simulink model "twolinkDynamics"  (R2017b)
settings: Solver=VariableStepAuto  StartTime=0.0  StopTime=360  RelTol=1e-3
libraries: simulink x1
settings Model: SimulationMode=accelerator  Creator=ArsalanBangash  LastModifiedBy=ArsalanBangash

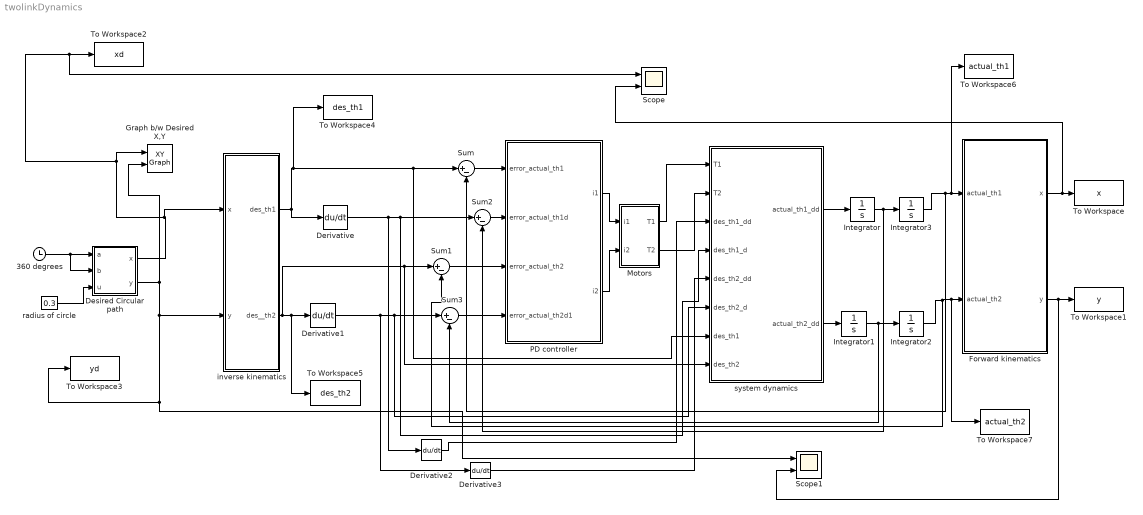
== system twolinkDynamics ==
  360 degrees : Clock
      settings: Decimation=360
  Derivative{,1..3} (4 alike) : Derivative
  Desired Circular path : MATLAB Function  TreatAsAtomicUnit=on
  "Forward kinematics " : MATLAB Function  TreatAsAtomicUnit=on
  Graph b/w Desired X,Y : simulink/Sinks/XY Graph  xmin=0  xmax=2  ymin=0  ymax=2  st=1
  Integrator{,1..3} (4 alike) : Integrator
  "Motors " : MATLAB Function  TreatAsAtomicUnit=on
  PD controller : Subsystem
  Scope : Scope  NumInputPorts=2
  Scope1 : Scope  NumInputPorts=2
  Sum{,1..3} (4 alike) : Sum  Inputs=|+-
  To Workspace : ToWorkspace  VariableName=x  SampleTime=1
  To Workspace1 : ToWorkspace  VariableName=y  SampleTime=1
  To Workspace2 : ToWorkspace  VariableName=xd  SampleTime=-1
  To Workspace3 : ToWorkspace  VariableName=yd  SampleTime=-1
  To Workspace4 : ToWorkspace  VariableName=des_th1  SampleTime=-1
  To Workspace5 : ToWorkspace  VariableName=des_th2  SampleTime=-1
  To Workspace6 : ToWorkspace  VariableName=actual_th1  SampleTime=-1
  To Workspace7 : ToWorkspace  VariableName=actual_th2  SampleTime=-1
  inverse kinematics : MATLAB Function  TreatAsAtomicUnit=on
  radius of circle : Constant  Value=0.3
  system dynamics : MATLAB Function  TreatAsAtomicUnit=on
  wires:
  360 degrees/1 -> Desired Circular path/2(b), Desired Circular path/1(a)
  radius of circle/1 -> Desired Circular path/3(u)
  Desired Circular path/1(x) -> Scope/1, To Workspace2/1, Graph b/w Desired X,Y/1, inverse kinematics/1(x)
  inverse kinematics/1(des_th1) -> To Workspace4/1, system dynamics/7(des_th1), Sum/1, Derivative/1
  "Motors "/1(T1) -> system dynamics/1(T1)
  "Forward kinematics "/1(x) -> Scope/2, To Workspace/1
  "Forward kinematics "/2(y) -> Scope1/2, To Workspace1/1
  Sum/1 -> PD controller/1(error_actual_th1)
  Sum2/1 -> PD controller/2(error_actual_th1d)
  PD controller/1(i1) -> "Motors "/1(i1)
  PD controller/2(i2) -> "Motors "/2(i2)
  "Motors "/2(T2) -> system dynamics/2(T2)
  Sum1/1 -> PD controller/3(error_actual_th2)
  Sum3/1 -> PD controller/4(error_actual_th2d1)
  system dynamics/1(actual_th1_dd) -> Integrator/1
  Integrator/1 -> Sum2/2, Integrator3/1
  Integrator3/1 -> Sum/2, To Workspace6/1, "Forward kinematics "/1(actual_th1)
  system dynamics/2(actual_th2_dd) -> Integrator1/1
  Integrator1/1 -> Integrator2/1, Sum3/2
  Integrator2/1 -> To Workspace7/1, "Forward kinematics "/2(actual_th2), Sum1/2
  inverse kinematics/2(des__th2) -> To Workspace5/1, Derivative1/1, system dynamics/8(des_th2), Sum1/1
  Derivative/1 -> system dynamics/4(des_th1_d), Sum2/1, Derivative2/1
  Derivative3/1 -> system dynamics/5(des_th2_dd)
  Derivative2/1 -> system dynamics/3(des_th1_dd)
  Derivative1/1 -> Derivative3/1, system dynamics/6(des_th2_d), Sum3/1
  Desired Circular path/2(y) -> Scope1/1, To Workspace3/1, inverse kinematics/2(y), Graph b/w Desired X,Y/2

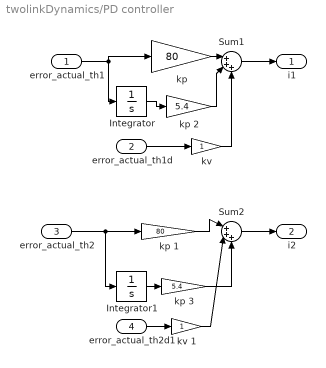
== system twolinkDynamics/PD controller ==
  error_actual_th1 : Inport
  error_actual_th1d : Inport  Port=2
  error_actual_th2 : Inport  Port=3
  error_actual_th2d1 : Inport  Port=4
  Integrator : Integrator
  Integrator1 : Integrator
  Sum1 : Sum  Inputs=|+++
  Sum2 : Sum  Inputs=|+++
  "kp " : Gain  Gain=80
  kp 1 : Gain  Gain=80
  kp 2 : Gain  Gain=5.4
  kp 3 : Gain  Gain=5.4
  "kv " : Gain
  kv 1 : Gain
  i1 : Outport
  i2 : Outport  Port=2
  wires:
  Sum1/1 -> i1/1
  "kp "/1 -> Sum1/1
  error_actual_th1d/1 -> "kv "/1
  error_actual_th1/1 -> Integrator/1, "kp "/1
  "kv "/1 -> Sum1/3
  error_actual_th2/1 -> Integrator1/1, kp 1/1
  kv 1/1 -> Sum2/2
  error_actual_th2d1/1 -> kv 1/1
  kp 1/1 -> Sum2/1
  Sum2/1 -> i2/1
  Integrator/1 -> kp 2/1
  kp 2/1 -> Sum1/2
  Integrator1/1 -> kp 3/1
  kp 3/1 -> Sum2/3

== matlab function twolinkDynamics/Motors  ==
  data: i1 input; T1 output; i2 input; T2 output
function [T1,T2]= fcn(i1,i2)
kt=10;
T1=kt*i1;
kt=10;
T2=kt*i2;

== matlab function twolinkDynamics/inverse kinematics ==
  data: x input; des_th1 output; y input; des__th2 output
function [des_th1,des__th2]= fcn(x,y)
L1=2;
L2=1;
M1=1;
M2=0.5;
c2= (x^2 +y^2 -L1^2 -L2^2)/(2*L1*L2)
s2=(1-c2^2)^0.5
K1= L1+L2*c2
K2=L2*s2
des_th1= atan2 (y,x)-atan2(K2,K1);
des__th2=atan2 (s2,c2);

== matlab function twolinkDynamics/Desired Circular path ==
  data: x output; a input; y output; b input; u input
function [x,y]= fcn(a,b,u)


x= 1 +u*cosd(a);
y=1+u*sind(b);

== matlab function twolinkDynamics/system dynamics ==
  data: T1 input; actual_th1_dd output; T2 input; actual_th2_dd output; des_th1_dd input; des_th1_d input; des_th2_dd input; des_th2_d input; des_th1 input; des_th2 input
function [actual_th1_dd,actual_th2_dd]= fcn(T1, T2,des_th1_dd,des_th1_d,des_th2_dd,des_th2_d,des_th1,des_th2)



N=1;
jm1=0.01;
jm2=0.01;
cm1=0.1;
cm2=0.1;
M1=1;
M2=0.5;
L1=2;
L2=1;
g=9.8;

th1=des_th1
th2=des_th2
th1dd=des_th1_dd
th1d=des_th1_d
th2dd=des_th2_dd
th2d=des_th2_d

M=[((M1+M2)*(L1^2)+ (M2*L2^2)+ (2*M2*L1*L2*cos(th2)))  (M2*L2^2+ M2*L1*L2*cos(th2));
   (M2*L2^2+M2*L1*L2*cos(th2))                   (M2*L2^2)];


V=[((-M2*L1*L2)*(2*th1d*th2d+th2d^2)*sin(th2));
   (M2*L1*L2*th1d^2*sin(th2))];




 G= [((M1+M2)*g*L1*cos(th1)+M2*g*L2*cos(th1+th2));
     M2*g*L2*cos(th1+th2)];
 
 Tt1= N*T1 -N^2* jm1*des_th1_dd -N^2*cm1 *des_th1_d
 Tt2= N*T2 -N^2* jm2*des_th2_dd -N^2*cm2 *des_th2_d
 
NJ=[N*jm1 0;
   0 N*jm2]

NT=[N*T1;
N*T2]

NC=[N*cm1 0;
0 N*cm2]

thd=[des_th1_d;
des_th1_d]


actual_th_dd= inv(M+NJ) *(NT -V- G-(NC*thd));
v= actual_th_dd(1)
w=actual_th_dd(2)

actual_th1_dd=v
actual_th2_dd=w

== matlab function twolinkDynamics/Forward kinematics  ==
  data: x output; actual_th1 input; y output; actual_th2 input
function [x,y]= fcn(actual_th1,actual_th2)

L1=2;
L2=1;


x=L2*cos(actual_th1 + actual_th2) + L1*cos(actual_th1)
y=L2*sin(actual_th1 + actual_th2) + L1*sin(actual_th1)
